simulink model "Modelo2020a"  (R2020a)
settings: Solver=FixedStepAuto  StartTime=0.0  StopTime=inf  FixedStep=5e-4  MaxStep=1e-4  RelTol=1e-3
model workspace (MAT data in the model file):
  sensor_carga : Simulink.Parameter (value not decoded)
values from neighbouring files (symbols this model uses):
  bcx = 1000e3    (= 1000000)    [Datos_simulacion.m]
  bcy = 500e3    (= 500000)    [Datos_simulacion.m]
  beq_tc = (bv_c+beq_cel)/Rw^2    (= 27000)    [Datos_simulacion.m]
  beq_ti = (b_h+beq_iel)/Rd^2    (= 28800)    [Datos_simulacion.m]
  bw = 30e3    (= 30000)    [Datos_simulacion.m]
  g = 9.80665    [Datos_simulacion.m]
  i_c = 15    [Datos_simulacion.m]
  i_i = 30    [Datos_simulacion.m]
  Kcd = Meq_c*polo_c*n    (= 472500)    [Datos_simulacion.m]
  Kci = Kcp*polo_c/n    (= 1938936.66179)    [Datos_simulacion.m]
  Kcp = Kcd*polo_c    (= 1513396.48861)    [Datos_simulacion.m]
  Kcy = 1.3e9    (= 1300000000)    [Datos_simulacion.m]
  Kid = Kcp*polo_i/n    (= 1815537.84919)    [Datos_simulacion.m]
  Kii = Meq_i*polo_i*n    (= 360000)    [Datos_simulacion.m]
  Kip = Kcd*polo_i    (= 1417080.12441)    [Datos_simulacion.m]
  Kw = 1800e3    (= 1800000)    [Datos_simulacion.m]
  Meq_c = m_c+Jeq_c/Rw^2    (= 59008)    [Datos_simulacion.m]
  Meq_i = m_h+Jeq_i/Rd^2    (= 48014.2222222)    [Datos_simulacion.m]
  Rd = 0.75    [Datos_simulacion.m]
  Rw = 0.5    [Datos_simulacion.m]
  Tau = 1e-3    (= 0.001)    [Datos_simulacion.m]
undefined symbols (not defined in the file or in its folder): DiscIntNeverNeededParam
libraries: simulink x4, fuzblock x1, dspswit3 x1, powerlib_meascontrol x1, dspfdesign x1
(part 2 of 2)

== stateflow chart Modelo2020a/NIVEL 0 ==
  state NORMAL
    state WATCHDOG [parallel]
      en:
      alarmaM=0;
      du:
      if(S_e1==0)
      alarmaM=1;
      end
      if(S_e2==0)
      alarmaM=1;
      end
      if(S_e3==0)
      alarmaM=1;
      end
      settings: executionOrder=2
    state CHEQUEO_ERROR [parallel]
      settings: executionOrder=1
      state Normal
        en:flag_emergencia=0;
        alarmaIz=0;
        alarmaC=0;
        alarmaG=0;
        flag_control=0;
      state ErrorIzaje
        en :
        alarmaIz=1;
      state ErrorCarro
        alarmaC=1;
      state ErrorGeneral
        alarmaG=1;
      (default) -> Normal
      Normal -> ErrorIzaje [order 1] : [FCi||vMi<vi]
      Normal -> ErrorCarro [order 2] : [FCxc_80 || FCxc_0 || vc>4]
      ErrorIzaje -> ErrorGeneral : [[FCxc_80 || FCxc_0 || vc>4]]
      ErrorCarro -> ErrorGeneral : [[FCi||vMi<vi]]
  state EMERGENCIA
    state ReduVeltransicion1
      en:
      flag_control=1;
      time_a=time;
      delta_t=0;
      vx=vc;
      vy=vi;
      du:
      delta_t=time-time_a;
      [vx,vy]=Calc_v1(delta_t,vx,vy)
      time_a=time;
      ex:
      vx = 0
      vy = 0
    state EstadoManual
      en :
      time_a=time;
      vx_a=0;
      vy_a=0;
      delta_t=0;
      flag_emergencia=1;
      du :
      delta_t=time-time_a;
      [vx,vy]=Calc_v(delta_t,vx_a,vy_a,X_com,Y_com);
      time_a=time;
      vx_a=vx;
      vy_a=vy;
    state Apagar_alarm
      en:
      alarmaIz=0;
      alarmaC=0;
      alarmaG=0;
      alarmaM=0
    (default) -> ReduVeltransicion1
    ReduVeltransicion1 -> EstadoManual : [abs(vx)<0.1 && abs(vy)<0.01 && theta<0.05]
    EstadoManual -> Apagar_alarm : [FinEmer]
  (default) -> NORMAL
  NORMAL -> EMERGENCIA : [alarmaM||alarmaG||alarmaC||alarmaIz]
  EMERGENCIA -> NORMAL : [alarmaM==0&&alarmaG==0&&alarmaC==0&&alarmaIz==0]
  data: delta_t2 function_input double; vx_a2 function_input double; vy_a2 function_input double; vx2 function_output; vy2 function_output; delta_t1 function_input double; vx_a1 function_input double; vy_a1 function_input double; vx1 function_output; vy1 function_output; X_com1 function_input; Y_com1 function_input; FCxc_80 input; FCxc_0 input; FCi input; S_e1 input; S_e2 input; S_e3 input; vMi input; vi input; vc input; time input; X_com input; Y_com input; yCarro_pos input; alarmaC output; alarmaG output; alarmaIz output; alarmaM output; time_a local; vx_a local; vy_a local; delta_t local; vy output; vx output; FinEmer input; flag_control output; flag_emergencia output; theta input
  function [vx2,vy2]=Calc_v1(delta_t2,vx_a2,vy_a2):
    | function [vx2,vy2]=Calc_v1(delta_t2,vx_a2,vy_a2)
    | if (vx_a2 < 0 )
    |     vx2=0.2*(delta_t2)+vx_a2;
    | else
    |     vx2=-0.2*(delta_t2)+vx_a2;
    | end
    | if (vy_a2 < 0)
    |     vy2=0.2*(delta_t2)+vy_a2
    | else
    |     vy2=-0.2*(delta_t2)+vy_a2
    | end
    | end
  function [vx1,vy1]=Calc_v(delta_t1,vx_a1,vy_a1,X_com1,Y_com1):
    | function [vx1,vy1]=Calc_v(delta_t1,vx_a1,vy_a1,X_com1,Y_com1)
    | if (X_com1 == 29 && vx_a1<4)
    |     vx1=0.8*(delta_t1)+vx_a1;
    | elseif (X_com1 == 28 && vx_a1 > -4 )
    |     vx1=-0.8*(delta_t1)+vx_a1;
    | else
    |     vx1=vx_a1;
    | end
    | if (Y_com1 == 31 && vy_a1<1.5)
    |     vy1=0.8*(delta_t1)+vy_a1
    | elseif (Y_com1==30 && vy_a1>-1.5)
    |     vy1=-0.8*(delta_t1)+vy_a1
    | else
    |     vy1=vy_a1
    | end
    | 
    | end

== matlab function Modelo2020a/Position_dump/MATLAB Function ==
  data: qd input size=2,1000000; cont_i input; vt output; vi output
 function [vt,vi] = fcn(qd,cont_i)
 cont_i=int32(cont_i);
 if (cont_i<length(qd(1,:)))
   cont=cont_i+1;
   vt = qd(1,cont);
   vi = qd(2,cont);
 else
  vt = 0;
  vi = 0;
 end
 
 end

== matlab function Modelo2020a/Busqueda de camino y interpolacion/Interpolador ==
  data: wayPoints input size=2,100; q output size=[2,1000000]; velMaxX input; velMaxY input
function q  = Interp(wayPoints,velMaxX,velMaxY)
coder.extrinsic('plot')
pendiente_ant=-nan;
cont_p=1;
wayPoints=wayPoints([2,1],:)
wayPoints=flip(wayPoints,2)
wayPoints(2,:)=(wayPoints(2,:)-65)*-1
for i=1:length(wayPoints)-1
    pendiente=(wayPoints(2,i)-wayPoints(2,i+1))/(wayPoints(1,i)-wayPoints(1,i+1));
    if pendiente_ant~=pendiente
        cont_p=cont_p+1;
    end
    pendiente_ant=pendiente;
end
wayPoints1=zeros(2,cont_p);
cont_p2=0;
for i=1:length(wayPoints(1,:))-1
    pendiente=(wayPoints(2,i)-wayPoints(2,i+1))/(wayPoints(1,i)-wayPoints(1,i+1));
    if pendiente_ant~=pendiente
    cont_p2=cont_p2+1;
    wayPoints1(:,cont_p2)=wayPoints(:,i);
    end
    pendiente_ant=pendiente;
end
wayPoints1(:,end)=wayPoints(:,end);
wayPoints1(:,1)=wayPoints(:,1);
figure(10)
plot(wayPoints1(1,:),wayPoints1(2,:))   
vx_max=velMaxX;
vy_max=velMaxY;
timePoints1=zeros(1,length(wayPoints1));
tiempo_ant=0;
for i=1:length(wayPoints1(1,:))-1
    restaX=abs(wayPoints1(1,i+1)-wayPoints1(1,i));
    restaY=abs(wayPoints1(2,i+1)-wayPoints1(2,i));
    timex=restaX/(vx_max/2.5);
    timey=restaY/(vy_max/2.5);
    if timex>timey
    timePoints1(i+1)=restaX/(vx_max/4)+tiempo_ant;
    elseif timex<timey
    timePoints1(i+1)=restaY/(vy_max/4)+tiempo_ant;
    else
     timePoints1(i+1)=restaX/(vx_max/4)+tiempo_ant;    
    end
    tiempo_ant=timePoints1(i+1);
end
tSamples1=0:5e-4:timePoints1(end);
q = zeros(2,length(tSamples1));%'VelocityBoundaryCondition',vel_max);
qx=interp1(timePoints1,wayPoints1(1,:),tSamples1,'pchip');
qy=interp1(timePoints1,wayPoints1(2,:),tSamples1,'pchip');
q(1,:)=qx;
q(2,:)=qy;
figure(15)
plot(qx,qy)  

end

== matlab function Modelo2020a/Modelo de planta/Piso/MATLAB Function ==
  data: u input; y output
function y = fcn(u)
if u>30
    y=0;
else 
    y=20;
end
